simulink library "MeasuringLibrary"  (R2021a)
settings: Solver=VariableStepAuto  StartTime=0.0  StopTime=10.0  RelTol=1e-3
libraries: simulink x5, $bdroot x4
settings Model: Creator=phill  LastModifiedBy=phill

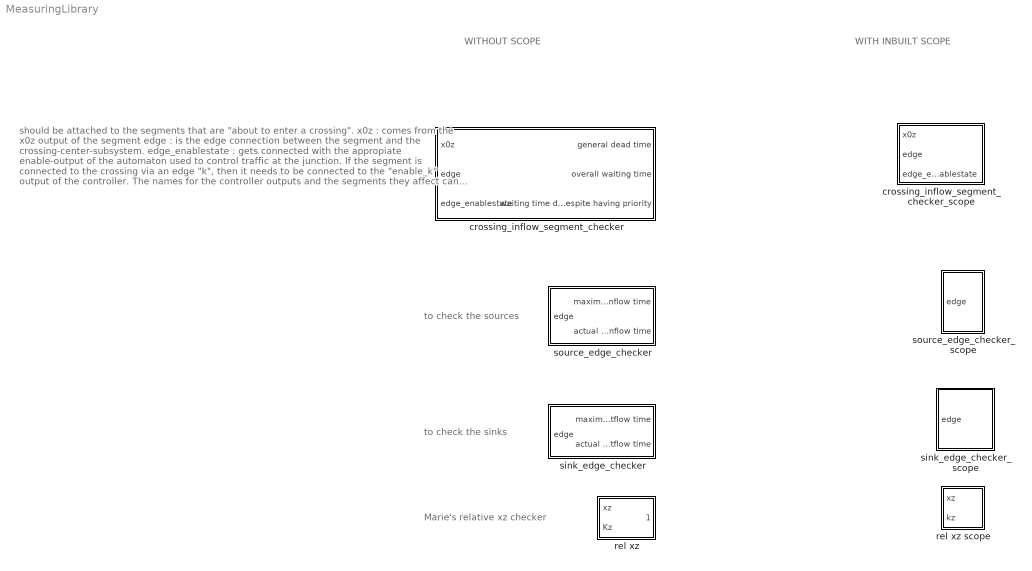
== system MeasuringLibrary ==
  note: to check the sources
  note: WITHOUT SCOPE
  note: should be attached to the segments that are "about to enter a crossing".
      | x0z : comes from the x0z output of the segment
      | edge : is the edge connection between the segment and the crossing-center-subsystem.
      | edge_enablestate : gets connected with the appropiate enable-output of the automaton
      | used to control traffic at the junction. If the segment is connected to the crossing via an edge "k", then it needs to be connected to the "enable_k" output of the controller.
      | The names for the controller outputs and the segments they affect can be taken
      | from screenshots in our documentation. (careful with the rotated T crossing here!)
      |
      | might be a good idea to use goto/from blocks to connect the controller to this subsystem
  note: WITH INBUILT SCOPE
  note: to check the sinks
  note: Marie's relative xz
      | checker
  crossing_inflow_segment_checker : Subsystem
  crossing_inflow_segment_checker_scope : Subsystem
  rel xz : Subsystem
  rel xz scope : Subsystem
  sink_edge_checker : Subsystem  mask{shortestPathTz=0}
      mask prompts: shortestPathTz "Sum of Tz on the path to the closest source"
      mask Display: disp(['pathTz = ', get_param(gcb,'shortestPathTz')])
  sink_edge_checker_scope : Subsystem  mask{shortestPathTz=0}
      mask prompts: shortestPathTz "Sum of Tz on the path to the closest source"
      mask Display: disp(['pathTz = ', get_param(gcb,'shortestPathTz')])
  source_edge_checker : Subsystem
  source_edge_checker_scope : Subsystem

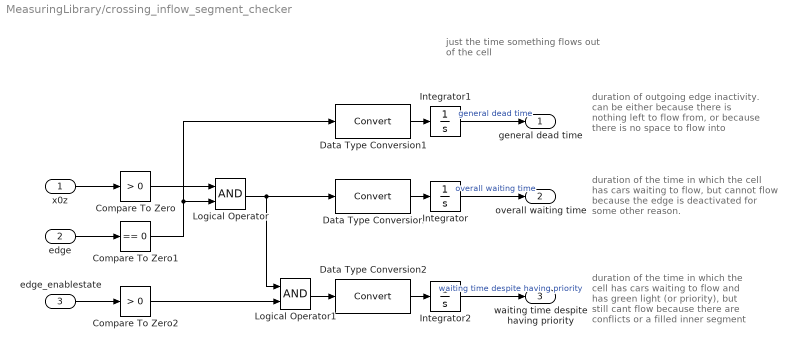
== system MeasuringLibrary/crossing_inflow_segment_checker ==
  note: just the time something flows out
      | of the cell
  note: duration of the time in which
      | the cell has cars waiting to flow,
      | but cannot flow because the edge
      | is deactivated for some other reason.
  note: duration of outgoing edge inactivity.
      | can be either because
      | there is nothing left to flow
      | from, or because there is no
      | space to flow into
  note: duration of the time in which
      | the cell has cars waiting to flow
      | and has green light (or priority),
      | but still cant flow because there
      | are conflicts or a filled inner
      | segment
  x0z : Inport
  edge : Inport  Port=2
  edge_enablestate : Inport  Port=3
  Compare To Zero : simulink/Logic and Bit Operations/Compare To Zero  relop=>  OutDataTypeStr=boolean
  Compare To Zero1 : simulink/Logic and Bit Operations/Compare To Zero  relop===  OutDataTypeStr=boolean
  Compare To Zero2 : simulink/Logic and Bit Operations/Compare To Zero  relop=>  OutDataTypeStr=boolean
  Data Type Conversion : DataTypeConversion
  Data Type Conversion1 : DataTypeConversion
  Data Type Conversion2 : DataTypeConversion
  Integrator : Integrator
  Integrator1 : Integrator
  Integrator2 : Integrator
  Logical Operator : Logic  AllPortsSameDT=off  OutDataTypeStr=boolean
  Logical Operator1 : Logic  AllPortsSameDT=off  OutDataTypeStr=boolean
  general dead time : Outport
  overall waiting time : Outport  Port=2
  waiting time despite having priority : Outport  Port=3
  wires:
  x0z/1 -> Compare To Zero/1
  Integrator/1 -> overall waiting time/1  "overall waiting time"
  edge/1 -> Compare To Zero1/1
  Logical Operator/1 -> Logical Operator1/1, Data Type Conversion/1
  Data Type Conversion/1 -> Integrator/1
  Compare To Zero/1 -> Logical Operator/1
  Integrator2/1 -> waiting time despite having priority/1  "waiting time despite having priority"
  Integrator1/1 -> general dead time/1  "general dead time"
  Compare To Zero2/1 -> Logical Operator1/2
  Data Type Conversion1/1 -> Integrator1/1
  Compare To Zero1/1 -> Data Type Conversion1/1, Logical Operator/2
  edge_enablestate/1 -> Compare To Zero2/1
  Logical Operator1/1 -> Data Type Conversion2/1
  Data Type Conversion2/1 -> Integrator2/1

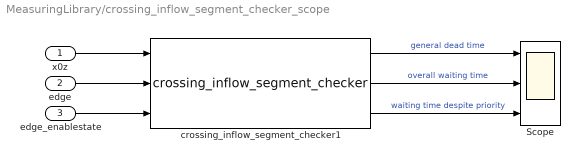
== system MeasuringLibrary/crossing_inflow_segment_checker_scope ==
  x0z : Inport
  edge : Inport  Port=2
  edge_enablestate : Inport  Port=3
  Scope : Scope  NumInputPorts=3
  crossing_inflow_segment_checker1 : $bdroot/crossing_inflow_segment_checker  SystemSampleTime=-1  VariantActivationTime=update diagram  Latency=0  AutoFrameSizeCalculation=off
  wires:
  crossing_inflow_segment_checker1/1 -> Scope/1  "general dead time"
  edge_enablestate/1 -> crossing_inflow_segment_checker1/3
  crossing_inflow_segment_checker1/2 -> Scope/2  "overall waiting time"
  edge/1 -> crossing_inflow_segment_checker1/2
  x0z/1 -> crossing_inflow_segment_checker1/1
  crossing_inflow_segment_checker1/3 -> Scope/3  "waiting time despite priority"

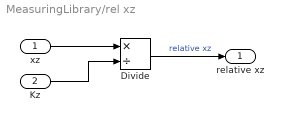
== system MeasuringLibrary/rel xz ==
  xz : Inport
  Kz : Inport  Port=2
  Divide : Product  Inputs=*/
  relative xz : Outport
  wires:
  Kz/1 -> Divide/2
  Divide/1 -> relative xz/1  "relative xz"
  xz/1 -> Divide/1

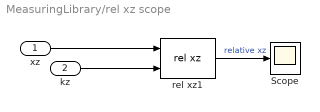
== system MeasuringLibrary/rel xz scope ==
  xz : Inport
  kz : Inport  Port=2
  Scope : Scope
  rel xz1 : $bdroot/rel xz  SystemSampleTime=-1  VariantActivationTime=update diagram  Latency=0  AutoFrameSizeCalculation=off
  wires:
  kz/1 -> rel xz1/2
  rel xz1/1 -> Scope/1  "relative xz"
  xz/1 -> rel xz1/1

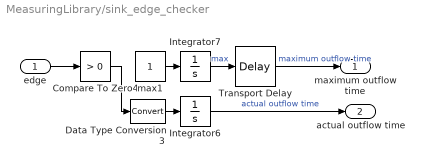
== system MeasuringLibrary/sink_edge_checker ==
  edge : Inport
  Compare To Zero4 : simulink/Logic and Bit Operations/Compare To Zero  relop=>  OutDataTypeStr=uint8
  Data Type Conversion3 : DataTypeConversion
  Integrator6 : Integrator
  Integrator7 : Integrator
  Transport Delay : TransportDelay  DelayTime=shortestPathTz
  max1 : Constant
  maximum outflow time : Outport
  actual outflow time : Outport  Port=2
  wires:
  Transport Delay/1 -> maximum outflow time/1  "maximum outflow time"
  Integrator7/1 -> Transport Delay/1  "max"
  Integrator6/1 -> actual outflow time/1  "actual outflow time"
  Compare To Zero4/1 -> Data Type Conversion3/1
  edge/1 -> Compare To Zero4/1
  Data Type Conversion3/1 -> Integrator6/1
  max1/1 -> Integrator7/1

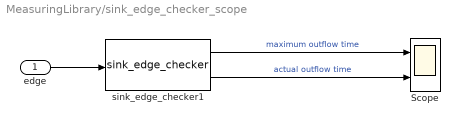
== system MeasuringLibrary/sink_edge_checker_scope ==
  edge : Inport
  Scope : Scope  NumInputPorts=2
  sink_edge_checker1 : $bdroot/sink_edge_checker  shortestPathTz=shortestPathTz
  wires:
  sink_edge_checker1/2 -> Scope/2  "actual outflow time"
  edge/1 -> sink_edge_checker1/1
  sink_edge_checker1/1 -> Scope/1  "maximum outflow time"

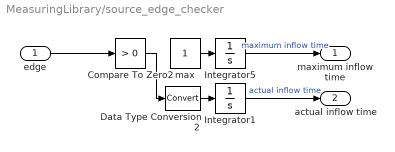
== system MeasuringLibrary/source_edge_checker ==
  edge : Inport
  Compare To Zero2 : simulink/Logic and Bit Operations/Compare To Zero  relop=>  OutDataTypeStr=uint8
  Data Type Conversion2 : DataTypeConversion
  Integrator1 : Integrator
  Integrator5 : Integrator
  max : Constant
  maximum inflow time : Outport
  actual inflow time : Outport  Port=2
  wires:
  Integrator5/1 -> maximum inflow time/1  "maximum inflow time"
  max/1 -> Integrator5/1
  edge/1 -> Compare To Zero2/1
  Data Type Conversion2/1 -> Integrator1/1
  Compare To Zero2/1 -> Data Type Conversion2/1
  Integrator1/1 -> actual inflow time/1  "actual inflow time"

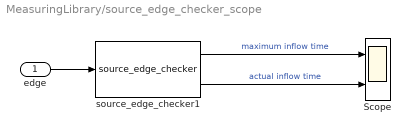
== system MeasuringLibrary/source_edge_checker_scope ==
  edge : Inport
  Scope : Scope  NumInputPorts=2
  source_edge_checker1 : $bdroot/source_edge_checker  SystemSampleTime=-1  VariantActivationTime=update diagram  Latency=0  AutoFrameSizeCalculation=off
  wires:
  edge/1 -> source_edge_checker1/1
  source_edge_checker1/2 -> Scope/2  "actual inflow time"
  source_edge_checker1/1 -> Scope/1  "maximum inflow time"
